simulink model "tire_model_s"  (R2018b)
settings: Solver=VariableStepAuto  StartTime=0.0  StopTime=10.0  RelTol=1e-3
values from neighbouring files (symbols this model uses):
  A = 2    [tire_model.m]
  b_a = 0.8    [tire_model.m]
  C_d = 0.82    [tire_model.m]
  M = 300*kg    (= 300)    [tire_model.m]
  P_2_0 = 0    [tire_model.m]
  r = 0.3    [tire_model.m]
  rho = 1.225    [tire_model.m]
  Ts = Tfin/Nr_Ts_Points    (= 0.005)    [tire_model.m]
libraries: simulink x1
settings Model: Creator=annac  LastModifiedBy=annac

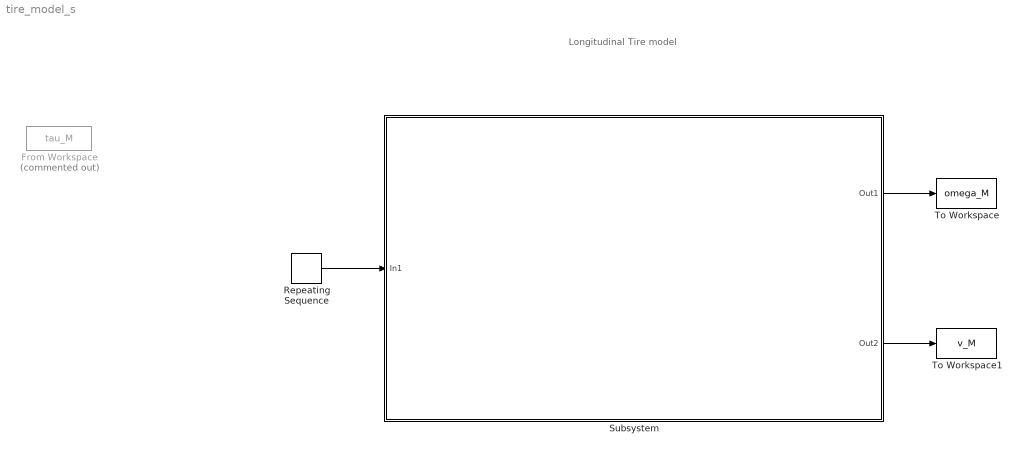
== system tire_model_s ==
  note: Longitudinal Tire model
  From Workspace : FromWorkspace  Commented=on  VariableName=tau_M  SampleTime=0
  Repeating Sequence : simulink/Sources/Repeating Sequence  rep_seq_t=[0 5 7 10]  rep_seq_y=[0 1000 3000 10000]
  Subsystem : Subsystem
  To Workspace : ToWorkspace  VariableName=omega_M  SampleTime=-1
  To Workspace1 : ToWorkspace  VariableName=v_M  SampleTime=-1
  wires:
  Subsystem/1(Out1) -> To Workspace/1
  Subsystem/2(Out2) -> To Workspace1/1
  Repeating Sequence/1 -> Subsystem/1(In1)

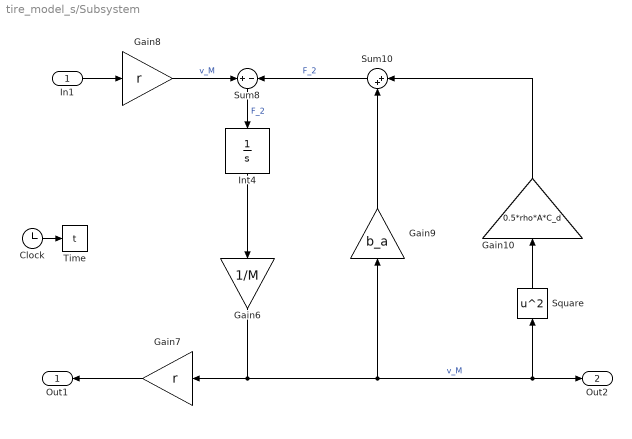
== system tire_model_s/Subsystem ==
  In1 : Inport
  Clock : Clock
  Gain10 : Gain  Gain=0.5*rho*A*C_d  SaturateOnIntegerOverflow=on  OutDataTypeStr=Inherit: Same as input  ParamDataTypeStr=Inherit: Same as input
  Gain6 : Gain  Gain=1/M  SaturateOnIntegerOverflow=on  OutDataTypeStr=Inherit: Same as input  ParamDataTypeStr=Inherit: Same as input
  Gain7 : Gain  Gain=r  SaturateOnIntegerOverflow=on  OutDataTypeStr=Inherit: Same as input  ParamDataTypeStr=Inherit: Same as input
  Gain8 : Gain  Gain=r  SaturateOnIntegerOverflow=on  OutDataTypeStr=Inherit: Same as input  ParamDataTypeStr=Inherit: Same as input
  Gain9 : Gain  Gain=b_a  SaturateOnIntegerOverflow=on  OutDataTypeStr=Inherit: Same as input  ParamDataTypeStr=Inherit: Same as input
  Int4 : Integrator  InitialCondition=P_2_0
  Square : Math  Operator=square  SaturateOnIntegerOverflow=on
  Sum10 : Sum  Inputs=|++  SaturateOnIntegerOverflow=on  InputSameDT=on  OutDataTypeStr=Inherit: Same as first input
  Sum8 : Sum  Inputs=+|-  SaturateOnIntegerOverflow=on  InputSameDT=on  OutDataTypeStr=Inherit: Same as first input
  Time : ToWorkspace  VariableName=t  SampleTime=Ts
      settings: MaxDataPoints=10000
  Out1 : Outport
  Out2 : Outport  Port=2
  wires:
  Gain7/1 -> Out1/1
  Gain8/1 -> Sum8/1  "v_M"
  Sum8/1 -> Int4/1  "F_2"
  Gain6/1 -> Gain7/1, Out2/1, Square/1, Gain9/1  "v_M"
  Int4/1 -> Gain6/1
  Gain10/1 -> Sum10/1
  Gain9/1 -> Sum10/2
  Sum10/1 -> Sum8/2  "F_2"
  Square/1 -> Gain10/1
  In1/1 -> Gain8/1
  Clock/1 -> Time/1
